simulink model "q4 - Kopya"  (R2018a)
settings: Solver=FixedStepDiscrete  StartTime=0  StopTime=0.6  FixedStep=1e-6  RelTol=1e-3
libraries: powerlib x19
settings Model: Creator=c  LastModifiedBy=asus

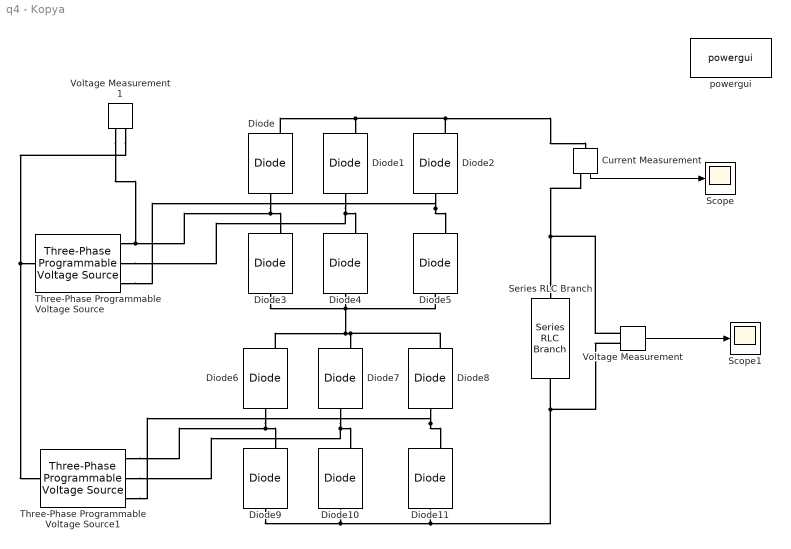
== system q4 - Kopya ==
  Current Measurement : powerlib/Measurements/Current Measurement  PhasorSimulation=off  OutputType=Complex  PSBequivalent=0
  Diode{,1..11} (12 alike) : powerlib/Power Electronics/Diode  Ron=1e-9  Lon=0  Vf=0  IC=0  UseSnubber=0  Rs=500  Cs=250e-9  Measurements=on
  Scope : Scope
  Scope1 : Scope
  Series RLC Branch : powerlib/Elements/Series RLC Branch  LConnTagsString=__new0  RConnTagsString=__new0  BranchType=R  Resistance=10  Inductance=1e-3  SetiL0=off  InitialCurrent=0  Capacitance=1e-6  Setx0=off  InitialVoltage=0  Measurements=None
  Three-Phase Programmable Voltage Source : powerlib/Electrical Sources/Three-Phase Programmable Voltage Source  PositiveSequence="[100  0 50]"  VariationEntity=None  VariationType=Table of time-amplitude pairs  VariationTypeAlt=Step  VariationStep=0.5  VariationRate=10  VariationMagnitude=0.3  VariationFrequency=2  VariationTiming=[1 2]  VariationPhaseA=off  Amplitudes=[1 0.8 1.2 1.0]  TimeValues=[0 0.1 0.15 0.2]  HarmonicGeneration=off  HarmonicA=[3 0.2 -25 0]  HarmonicB=[2 0.15 35 2]  Timing="[0.05  3]"  BusType=swing  Pref=0  Qref=0  Qmin=-inf  Qmax=inf
  Three-Phase Programmable Voltage Source1 : powerlib/Electrical Sources/Three-Phase Programmable Voltage Source  PositiveSequence="[100  30 50]"  VariationEntity=None  VariationType=Table of time-amplitude pairs  VariationTypeAlt=Step  VariationStep=0.5  VariationRate=10  VariationMagnitude=0.3  VariationFrequency=2  VariationTiming=[1 2]  VariationPhaseA=off  Amplitudes=[1 0.8 1.2 1.0]  TimeValues=[0 0.1 0.15 0.2]  HarmonicGeneration=off  HarmonicA=[3 0.2 -25 0]  HarmonicB=[2 0.15 35 2]  Timing="[0.05  3]"  BusType=swing  Pref=0  Qref=0  Qmin=-inf  Qmax=inf
  Voltage Measurement : powerlib/Measurements/Voltage Measurement  PhasorSimulation=off  OutputType=Complex  PSBequivalent=0
  Voltage Measurement1 : powerlib/Measurements/Voltage Measurement  PhasorSimulation=off  OutputType=Complex  PSBequivalent=0
  powergui : powerlib/powergui  Priority=1  SimulationMode=Discrete  SampleTime=5e-5  frequency=60  Iterations=50  frequencyindice=50  Pbase=100e6  ErrMax=1e-4  UnitsV=kV  UnitsW=MW  buscounter=0  FunctionMessages=off  echomessages=off  EnableUseOfTLC=off  CurrentSourceSwitches=off  DisableSnubberDevices=off  DisableRonSwitches=off  DisableVfSwitches=off  DisplayEquations=off  SolverType=Tustin/Backward Euler (TBE)  Interpol=off  ExternalGateDelay=off  methode=off  Ts=100  x0status=blocks  SPID=on  SwTol=0  HookPort=off  RestoreLinks=warning  ResistiveCurrentMeasurement=off  Frange=[0:2:500]  Ylog=off  Xlog=on  ShowGrid=off  save=off  variable=ZData  structure=0  ZoomFFT=off  StartTime=0.0  cycles=1  DisplayStyle=1  fundamental=60  FreqAxis=off  MaxFrequency=1000  frequencyindicesteady=1  RmsSteady=1  display=off
  wires:
  Current Measurement/1 -> Scope/1
  Voltage Measurement/1 -> Scope1/1
  connections:
  Diode/LConn1 -- Voltage Measurement1/LConn1 -- Three-Phase Programmable Voltage Source/RConn1 -- Diode3/RConn1
  Diode1/LConn1 -- Three-Phase Programmable Voltage Source/RConn2 -- Diode4/RConn1
  Diode2/LConn1 -- Diode5/RConn1 -- Three-Phase Programmable Voltage Source/RConn3
  Series RLC Branch/LConn1 -- Current Measurement/RConn1 -- Voltage Measurement/LConn1
  Diode6/LConn1 -- Three-Phase Programmable Voltage Source1/RConn1 -- Diode9/RConn1
  Diode9/LConn1 -- Diode10/LConn1 -- Voltage Measurement/LConn2 -- Series RLC Branch/RConn1 -- Diode11/LConn1
  Diode7/LConn1 -- Three-Phase Programmable Voltage Source1/RConn2 -- Diode10/RConn1
  Diode3/LConn1 -- Diode5/LConn1 -- Diode7/RConn1 -- Diode8/RConn1 -- Diode6/RConn1 -- Diode4/LConn1
  Diode8/LConn1 -- Three-Phase Programmable Voltage Source1/RConn3 -- Diode11/RConn1
  Diode2/RConn1 -- Current Measurement/LConn1 -- Diode/RConn1 -- Diode1/RConn1
  Voltage Measurement1/LConn2 -- Three-Phase Programmable Voltage Source1/LConn1 -- Three-Phase Programmable Voltage Source/LConn1
